simulink model "simulink_beliz"  (R2024b)
settings: Solver=VariableStepAuto  StartTime=0.0  StopTime=20  RelTol=1e-3
libraries: simulink x1
settings Model: PacingRate=10  Creator=ardaertanhan  LastModifiedBy=beliz
settings RTWCC: GPUComputeCapability=3.5

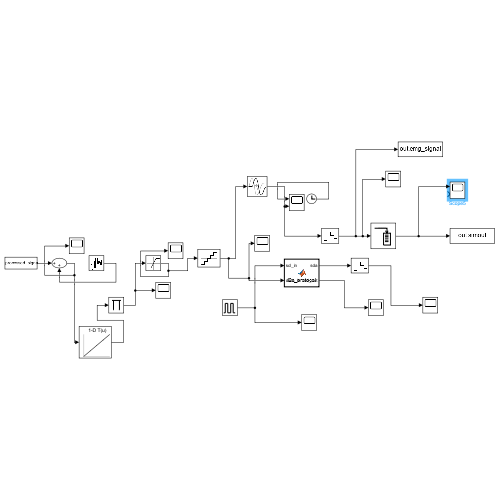
[thumbnail: Simulink's stored preview of the top-level diagram]
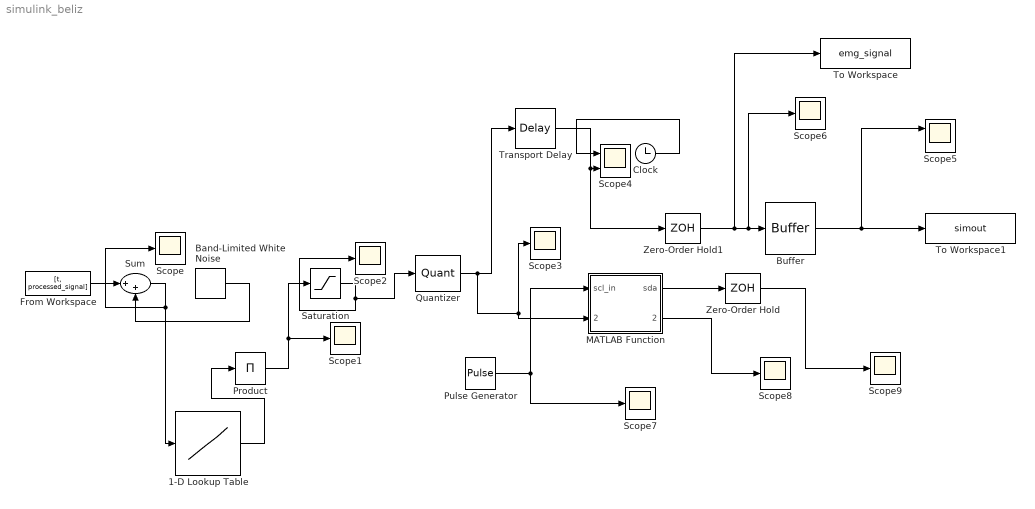
== system simulink_beliz ==
  1-D Lookup Table : Lookup_n-D  NumberOfTableDimensions=1  BreakpointsForDimension1=[-400, -200, 0, 200, 400]  Table=[1, 2, 3, 4, 5]  InternalRulePriority=Speed  RndMeth=Simplest
  Band-Limited White Noise : simulink/Sources/Band-Limited White Noise  Cov=[0.1]  Ts=0.1  seed=[23341]
  Buffer : Buffer  OutputFrames=off
  Clock : Clock
  From Workspace : FromWorkspace  VariableName=[t, processed_signal]  SampleTime=-1
  MATLAB Function : MATLAB Function  TreatAsAtomicUnit=on
  Product : Product  Inputs=1
  Pulse Generator : DiscretePulseGenerator  PulseType=Time based  Period=1e-5  PulseWidth=50
  Quantizer : Quantizer  QuantizationInterval=3 / 2^16
  Saturation : Saturate  UpperLimit=4.5  LowerLimit=1.5
  Scope{,1..3,6..9} (8 alike) : Scope
  Scope4 : Scope  NumInputPorts=2
  Scope5 : Scope  NumInputPorts=2
  Sum : Sum  Inputs=|++
  To Workspace : ToWorkspace  VariableName=emg_signal  SaveFormat=Timeseries  SampleTime=-1
  To Workspace1 : ToWorkspace  VariableName=simout  SaveFormat=Timeseries  SampleTime=-1
  Transport Delay : TransportDelay  DelayTime=2
  Zero-Order Hold : ZeroOrderHold  SampleTime=1 / 1000
  Zero-Order Hold1 : ZeroOrderHold  SampleTime=1e-3
  wires:
  From Workspace/1 -> Sum/1
  Band-Limited White Noise/1 -> Sum/2
  Sum/1 -> 1-D Lookup Table/1, Scope/1
  Saturation/1 -> Scope2/1, Quantizer/1
  Product/1 -> Saturation/1, Scope1/1
  Clock/1 -> Scope4/1
  Transport Delay/1 -> Zero-Order Hold1/1, Scope4/2
  Buffer/1 -> Scope5/1, To Workspace1/1
  Zero-Order Hold1/1 -> To Workspace/1, Scope6/1, Buffer/1
  1-D Lookup Table/1 -> Product/1
  Quantizer/1 -> Scope3/1, MATLAB Function/2(data_in), Transport Delay/1
  MATLAB Function/1(sda) -> Zero-Order Hold/1
  Pulse Generator/1 -> Scope7/1, MATLAB Function/1(scl_in)
  MATLAB Function/2(scl_out) -> Scope8/1
  Zero-Order Hold/1 -> Scope9/1

== matlab function simulink_beliz/MATLAB Function ==
  data: sda output; scl_in input; scl_out output; data_in input
function [sda, scl_out] = i2c_protocol(scl_in, data_in)
    % Inputs:
    % scl_in: Clock signal from Pulse Generator (double)
    % data_in: Data to transmit (vector of bytes, double but treated as uint8)
    %
    % Outputs:
    % sda: Simulated I²C data line (double)
    % scl_out: SCL signal passed through for visualization (double)

    % Persistent variables to retain state across clock cycles
    persistent sda_line bit_index byte_index transmitting last_scl;

    % Initialize persistent variables on first run
    if isempty(sda_line)
        sda_line = 1;          % SDA starts high (idle state)
        bit_index = 8;         % Start with the most significant bit (MSB)
        byte_index = 1;        % Start with the first byte in the data
        transmitting = false;  % Start in idle state
        last_scl = scl_in;     % Initialize clock state tracking
    end

    % Error handling: Check if data_in is empty
    if isempty(data_in)
        sda = 1;               % No data to send, SDA stays high
        scl_out = scl_in;      % Pass through the clock signal
        return;
    end

    % Error handling: Ensure byte_index doesn't exceed data_in size
    if byte_index > length(data_in)
        sda = 1;               % No more data to transmit, SDA stays high (idle)
        scl_out = scl_in;      % Pass through the clock signal
        return;
    end

    % Convert data_in to uint8 type, ensuring type consistency
    data_in = uint8(data_in);  % Convert to 8-bit unsigned integers

    % Explicitly declare outputs as double to avoid type mismatch in Simulink
    sda = double(sda_line);    % Default to the current SDA line state
    scl_out = double(scl_in);  % Pass the clock signal through unchanged

    % Detect rising and falling edges of scl_in
    rising_edge = (scl_in == 1) && (last_scl == 0);
    falling_edge = (scl_in == 0) && (last_scl == 1);

    % I²C Start Condition: Begin transmission when SCL is high and SDA falls
    if scl_in == 1 && sda_line == 1 && ~transmitting
        sda = 0;               % Pull SDA low to signal the start condition
        transmitting = true;   % Enter transmission state
        last_scl = scl_in;     % Update clock state
        return;                % Wait for next clock cycle
    end

    % I²C Data Transmission: Only change SDA on falling edges of SCL
    if falling_edge && transmitting
        if bit_index > 0
            % Extract the current bit to send
            sda = double(bitget(data_in(byte_index), bit_index));
            bit_index = bit_index - 1;  % Move to the next bit
        else
            % Move to the next byte when all bits of the current byte are sent
            bit_index = 8;             % Reset to MSB
            byte_index = byte_index + 1;
            
            % Check if all bytes have been transmitted
            if byte_index > length(data_in)
                sda = 1;               % Transmission complete, pull SDA high
                transmitting = false;  % Exit transmission state
                last_scl = scl_in;     % Update clock state
                return;
            end
        end
    end

    % I²C Stop Condition: Finish transmission when SCL is high and SDA rises
    if rising_edge && byte_index > length(data_in)
        sda = 1;               % Pull SDA high to signal the stop condition
        transmitting = false;  % Return to idle state
    end

    % Update persistent state
    sda_line = sda;            % Update SDA state
    last_scl = scl_in;         % Update clock state
end
